simulink model "FailureProcessing"  (R2014a)
settings: Solver=FixedStepDiscrete  StartTime=0.0  StopTime=SimLength  FixedStep=SampleTime  RelTol=1e-3
settings Model: Creator=georg  LastModifiedBy=Jonas
settings DataIOCC: MaxDataPoints=3000  ReturnWorkspaceOutputs=on

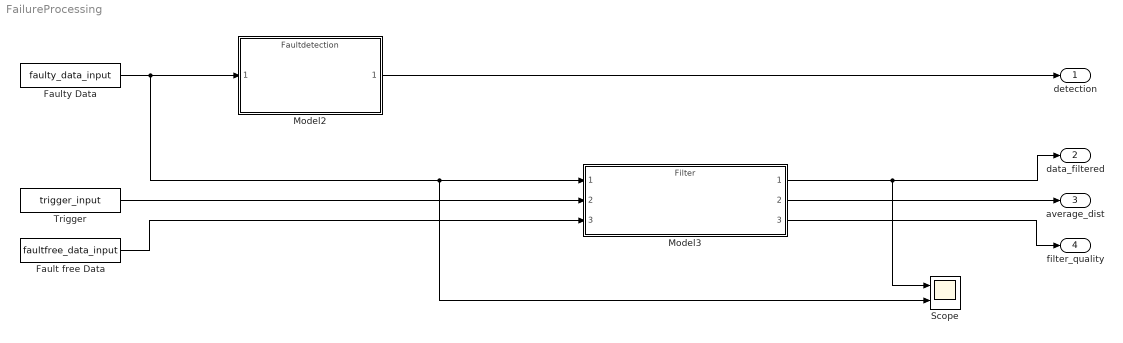
== system FailureProcessing ==
  Fault free Data : FromWorkspace  VariableName=faultfree_data_input  SampleTime=0
  Faulty Data : FromWorkspace  VariableName=faulty_data_input  SampleTime=0
  Model2 : ModelReference  ModelNameDialog=Faultdetection.slx  SimulationMode=Normal  ModelReferenceVersion=1.45  CopyOfModelName=Faultdetection.slx  DefaultDataLogging=on
  Model3 : ModelReference  ModelNameDialog=Filter  SimulationMode=Normal  ModelReferenceVersion=1.67  CopyOfModelName=Filter  DefaultDataLogging=on
  Scope : Scope  NumInputPorts=2
      settings: YMin=-5~-5  YMax=5~5
  Trigger : FromWorkspace  VariableName=trigger_input  OutDataTypeStr=Bus: TriggerBus  SampleTime=0
  detection : Outport
  data_filtered : Outport  Port=2
  average_dist : Outport  Port=3
  filter_quality : Outport  Port=4
  wires:
  Faulty Data/1 -> Model2/1, Scope/2, Model3/1
  Trigger/1 -> Model3/2
  Fault free Data/1 -> Model3/3
  Model2/1 -> detection/1
  Model3/1 -> Scope/1, data_filtered/1
  Model3/2 -> average_dist/1
  Model3/3 -> filter_quality/1
